simulink model "svm_tracking_1pred_sim"  (Simulink 8.6)
settings: Solver=VariableStepAuto  StartTime=0.0  StopTime=20  RelTol=1e-3
values from neighbouring files (symbols this model uses):
  K = ss(Ttuned.Blocks.K)    [svm_buildLinearControllers.m]
  My = ss(tf([eye(6) -eye(6)]))    [svm_buildLinearControllers.m]
  Mz = ss(tf([pickP, -pickP]))    [svm_buildLinearControllers.m]
  turbulence2loadfactors = blkdiag(T_w2nx, T_w2nz)    [svm_buildLinearControllers.m]
  uavsim = loaded.uavsim    [svm_sandbox.m]
  x0 = history(1).u_apst    [dsmc_extrinsic.m]    (also in svm_buildLinearControllers.m = [0 0 0 0 0 1 0 0 ])
undefined symbols (not defined in the file or in its folder): F, Light, MIL, sigbuilder_block, uavsimblockset_cartesianToAngle
libraries: aerolibwind2 x1, aerolibgravity2 x1, uavsimBlockset_VectorNorm x1, aerolibtransform2 x1
settings Model: Creator=j.bolting  LastModifiedBy=j.bolting
settings DataIOCC: SaveFormat=StructureWithTime  SignalLoggingSaveFormat=Dataset
settings OptimizationCC: BlockReduction=off  DefaultParameterBehavior=Inlined  BufferReuse=off  ExpressionDepthLimit=128
settings DebuggingCC: AlgebraicLoopMsg=none  UnderspecifiedInitializationDetection=Simplified  MergeDetectMultiDrivingBlocksExec=error  SolverPrmCheckMsg=none  FcnCallInpInsideContextMsg=EnableAllAsError  UnconnectedInputMsg=none  UnconnectedOutputMsg=none  UnconnectedLineMsg=none  StateNameClashWarn=none  InitInArrayFormatMsg=none
settings HardwareCC: ProdBitPerPointer=64  ProdLargestAtomicFloat=Float  ProdIntDivRoundTo=Zero  ProdEndianess=LittleEndian  ProdWordSize=64  ProdHWDeviceType=Intel->x86-64 (Windows64)
settings GRTTargetCC: GeneratePreprocessorConditionals=Use local settings  CombineOutputUpdateFcns=on  GRTInterface=off
settings ConfigComp: CovModelRefEnable=off

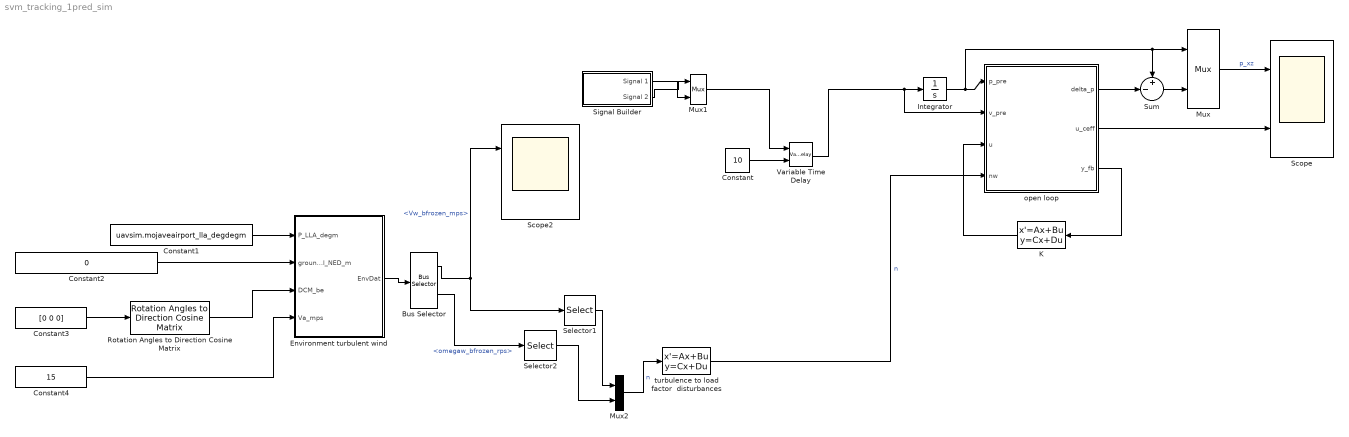
== system svm_tracking_1pred_sim ==
  Bus Selector : BusSelector  OutputSignals=Vw_bfrozen_mps,omegaw_bfrozen_rps
  Constant : Constant  Value=10
  Constant1 : Constant  Value=uavsim.mojaveairport_lla_degdegm
  Constant2 : Constant  Value=0
  Constant3 : Constant  Value=[0 0 0]
  Constant4 : Constant  Value=15
  Environment turbulent wind : Subsystem  AncestorBlock=uavsimBlockset_Environment_turbulentWind/Environment turbulent wind  mask{mask_constantwind_NED_mps=[5 0 0], mask_wingspan=uavsim.cularis.b, mask_windON=0, mask_turbulenceON=1}
      mask prompts: mask_constantwind_NED_mps "Ambient, i.e. constant wind vector [m/s], NED frame"; mask_wingspan "Aircraft wingspan"; mask_windON "Ambient wind ON?"; mask_turbulenceON "Turbulence ON?"
  Integrator : Integrator
  K : StateSpace  A=K.a  B=K.b  C=K.c  D=K.d  X0=0
  Mux : Mux  Inputs=2
  Mux1 : Mux  Inputs=2
  Mux2 : Mux  Inputs=2
  Rotation Angles to Direction Cosine Matrix : aerolibtransform2/Rotation Angles to Direction Cosine Matrix  rotationOrder=ZYX
  Scope : Scope  NumInputPorts=2
  Scope2 : Scope  NumInputPorts=2
  Selector1 : Selector  InputPortWidth=3  IndexOptions=Index vector (dialog)  Indices=[1 3]  OutputSizes=1
  Selector2 : Selector  InputPortWidth=3  IndexOptions=Index vector (dialog)  Indices=2  OutputSizes=1
  Signal Builder : Subsystem  Tag=STV Subsys  LoadFcn=sigbuilder_block('load');  StartFcn=sigbuilder_block('start');  StopFcn=sigbuilder_block('stop');  ClipboardFcn=sigbuilder_block('clipboard');  mask(Sigbuilder block){}
      mask help: Simulink:masks:SigbuilderBlock_MD
      mask init:
      | if ~strcmp(get_param(bdroot(gcbh),'SimulationStatus'),'stopped') tuvar = sigbuilder_block('maskInit'); end
      settings: CopyFcn=sigbuilder_block('copy');  DeleteFcn=sigbuilder_block('delete');  ModelCloseFcn=sigbuilder_block('modelClose');  PreSaveFcn=sigbuilder_block('preSave');  PauseFcn=sigbuilder_block('pause');  ContinueFcn=sigbuilder_block('continue');  NameChangeFcn=sigbuilder_block('namechange');  OpenFcn=sigbuilder_block('open',[437.6 199.2 550.4 400 ]);  CloseFcn=sigbuilder_block('close');
      mask Display: plot(0, 0, 100, 100,[2, 2, 32, 32, 2], [68, 8, 8, 68, 68],[32, 2], [38, 38], [32, 19, 2],[53, 60, 44], [32, 17, 17, 2],[16, 16, 31, 31]);txt = getActiveGroup(gcbh);text(2, 100, txt,'verticalAlignment', 'top');
  Sum : Sum  Inputs=+-|
  Variable Time Delay : VariableTransportDelay  MaximumDelay=1e3
  open loop : Subsystem
  turbulence to load factor  disturbances : StateSpace  A=turbulence2loadfactors.a  B=turbulence2loadfactors.b  C=turbulence2loadfactors.c  D=turbulence2loadfactors.d  X0=0
  wires:
  open loop/3(y_fb) -> K/1
  K/1 -> open loop/3(u)
  open loop/1(delta_p) -> Sum/2
  Sum/1 -> Mux/2
  Variable Time Delay/1 -> Integrator/1, open loop/2(v_pre)
  Mux/1 -> Scope/1  "p_xz"
  open loop/2(u_ceff) -> Scope/2
  Integrator/1 -> Sum/1, Mux/1, open loop/1(p_pre)
  Signal Builder/1(Signal 1) -> Mux1/2
  Signal Builder/2(Signal 2) -> Mux1/1
  Constant/1 -> Variable Time Delay/2
  Mux1/1 -> Variable Time Delay/1
  Environment turbulent wind/1(EnvDat) -> Bus Selector/1
  Bus Selector/1 -> Selector1/1, Scope2/1  "<Vw_bfrozen_mps>"
  Constant1/1 -> Environment turbulent wind/1(P_LLA_degm)
  Constant2/1 -> Environment turbulent wind/2(groundlevel_NED_m)
  Rotation Angles to Direction Cosine Matrix/1 -> Environment turbulent wind/3(DCM_be)
  Constant3/1 -> Rotation Angles to Direction Cosine Matrix/1
  Constant4/1 -> Environment turbulent wind/4(Va_mps)
  Bus Selector/2 -> Selector2/1  "<omegaw_bfrozen_rps>"
  Selector1/1 -> Mux2/1
  Selector2/1 -> Mux2/2
  Mux2/1 -> turbulence to load factor  disturbances/1  "n"
  turbulence to load factor  disturbances/1 -> open loop/4(nw)  "n"

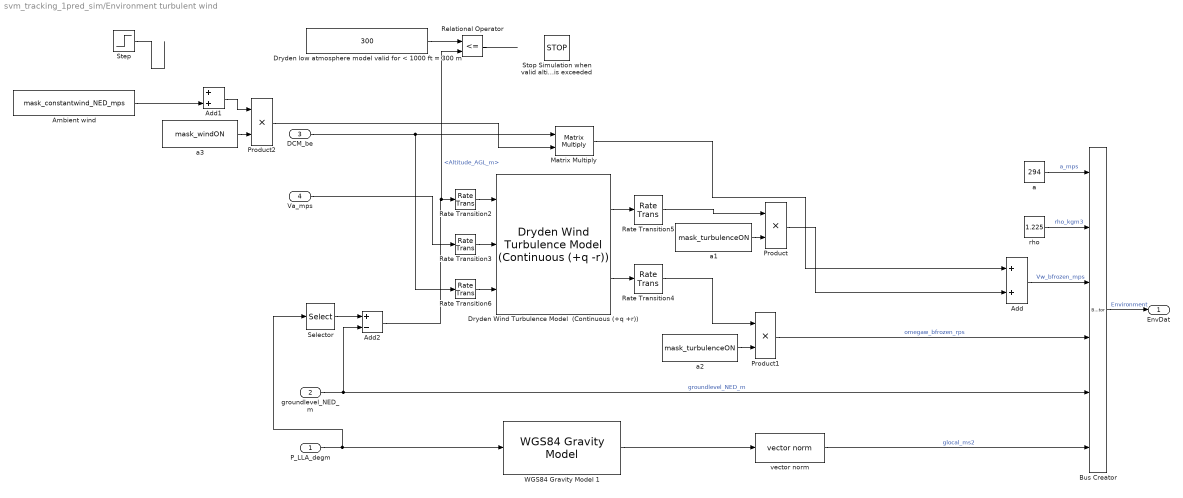
== system svm_tracking_1pred_sim/Environment turbulent wind ==
  P_LLA_degm : Inport
  groundlevel_NED_m : Inport  Port=2
  DCM_be : Inport  Port=3
  Va_mps : Inport  Port=4
  Add : Sum
  Add1 : Sum
  Add2 : Sum  Inputs=+-
  Ambient wind : Constant  Value=mask_constantwind_NED_mps
  Bus Creator : BusCreator  Inputs=6  OutDataTypeStr=Bus: Environment  NonVirtualBus=on
  Dryden Wind Turbulence Model  (Continuous (+q +r)) : aerolibwind2/Dryden Wind Turbulence Model  (Continuous (+q -r))  units=Metric (MKS)  spec=MIL-F-8785C  model=Discrete Dryden (+q -r)  W20=norm(mask_constantwind_NED_mps)  Wdeg=rad2deg(uavsimblockset_cartesianToAngle(mask_constantwind_NED_mps(1), mask_constantwind_NED_mps(2)))  TurbProb=10^-2 - Light  L_high=533.4  Wingspan=mask_wingspan  ts=0.1  Seed=randi(2^6, [1 4])  T_on=on
  Dryden low atmosphere model valid for < 1000 ft = 300 m : Constant  Value=300
  Matrix Multiply : Product  Multiplication=Matrix(*)
  Product : Product  RndMeth=Zero
  Product1 : Product  RndMeth=Zero
  Product2 : Product  RndMeth=Zero
  Rate Transition2 : RateTransition  OutPortSampleTime=0.1
  Rate Transition3 : RateTransition  OutPortSampleTime=0.1
  Rate Transition4 : RateTransition  OutPortSampleTime=0
  Rate Transition5 : RateTransition  OutPortSampleTime=0
  Rate Transition6 : RateTransition  OutPortSampleTime=0.1
  Relational Operator : RelationalOperator  Operator=<=  OutDataTypeStr=boolean
  Selector : Selector  InputPortWidth=3  IndexOptions=Index vector (dialog)  Indices=3  OutputSizes=1
  Step : Step  Time=10  After=[0 0 1]  SampleTime=0
  Stop Simulation when valid altitude is exceeded : Stop
  WGS84 Gravity Model 1 : aerolibgravity2/WGS84 Gravity Model   model=WGS84 Taylor Series  units=Metric (MKS)  no_atmos=on  precessing=on  jd_loc=off  month=October  day=10  year=2004  no_centrifugal=on  action=Warning
  a : Constant  Value=294
  a1 : Constant  Value=mask_turbulenceON
  a2 : Constant  Value=mask_turbulenceON
  a3 : Constant  Value=mask_windON
  "rho " : Constant  Value=1.225
  vector norm : uavsimBlockset_VectorNorm/vector norm
  EnvDat : Outport  OutDataTypeStr=Bus: Environment
  wires:
  Step/1 -> ?
  Add1/1 -> Product2/1
  Product2/1 -> Matrix Multiply/2
  a3/1 -> Product2/2
  Relational Operator/1 -> ?
  Dryden low atmosphere model valid for < 1000 ft = 300 m/1 -> Relational Operator/1
  Product1/1 -> Bus Creator/4  "omegaw_bfrozen_rps"
  a2/1 -> Product1/2
  a1/1 -> Product/2
  Product/1 -> Add/2
  Dryden Wind Turbulence Model  (Continuous (+q +r))/2 -> Rate Transition4/1
  P_LLA_degm/1 -> WGS84 Gravity Model 1/1, Selector/1
  groundlevel_NED_m/1 -> Add2/2, Bus Creator/5  "groundlevel_NED_m"
  WGS84 Gravity Model 1/1 -> vector norm/1
  Bus Creator/1 -> EnvDat/1  "Environment"
  "rho "/1 -> Bus Creator/2  "rho_kgm3"
  a/1 -> Bus Creator/1  "a_mps"
  Add/1 -> Bus Creator/3  "Vw_bfrozen_mps"
  vector norm/1 -> Bus Creator/6  "glocal_ms2"
  Add2/1 -> Rate Transition2/1, Relational Operator/2  "<Altitude_AGL_m>"
  Va_mps/1 -> Rate Transition3/1
  DCM_be/1 -> Matrix Multiply/1, Rate Transition6/1
  Ambient wind/1 -> Add1/2
  Dryden Wind Turbulence Model  (Continuous (+q +r))/1 -> Rate Transition5/1
  Matrix Multiply/1 -> Add/1
  Rate Transition4/1 -> Product1/1
  Rate Transition5/1 -> Product/1
  Selector/1 -> Add2/1
  Rate Transition2/1 -> Dryden Wind Turbulence Model  (Continuous (+q +r))/1
  Rate Transition3/1 -> Dryden Wind Turbulence Model  (Continuous (+q +r))/2
  Rate Transition6/1 -> Dryden Wind Turbulence Model  (Continuous (+q +r))/3

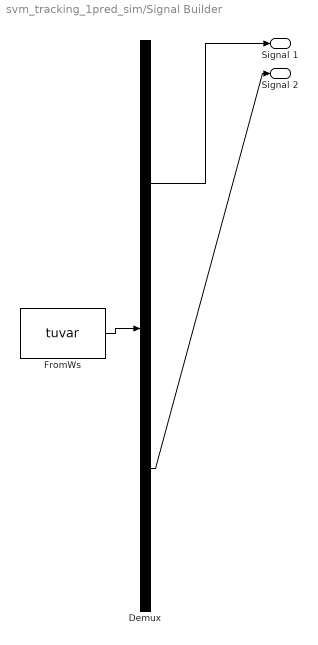
== system svm_tracking_1pred_sim/Signal Builder ==
  Demux : Demux  Tag=STV Demux  Outputs=2
  FromWs : FromWorkspace  Tag=STV FromWs  VariableName=tuvar  SampleTime=0  SigBuilderData=DataTag0  VnvData=DataTag1
      SigBuilderData=|
      | common.afterFinalStr = 'Extrapolate'
      | common.sampleTime = 0
      | dataSet.timeRange = [0 10]
      | dataSet.name = 'Group 1'
      | sbobj.Groups.Name = 'Group 1'
      | sbobj.Groups.Signals(1).Name = 'Signal 1'
      | sbobj.Groups.Signals(1).XData = [0 1.98 1.98 10]
      | sbobj.Groups.Signals(1).YData = [1 1 0 0.01]
      | sbobj.Groups.Signals(2).Name = 'Signal 2'
      | sbobj.Groups.Signals(2).XData = [0 4 6 10]
      | sbobj.Groups.Signals(2).YData = [0 0 0 0]
  Signal 1 : Outport  Tag=STV Outport
  Signal 2 : Outport  Tag=STV Outport  Port=2
  wires:
  Demux/1 -> Signal 1/1
  FromWs/1 -> Demux/1
  Demux/2 -> Signal 2/1

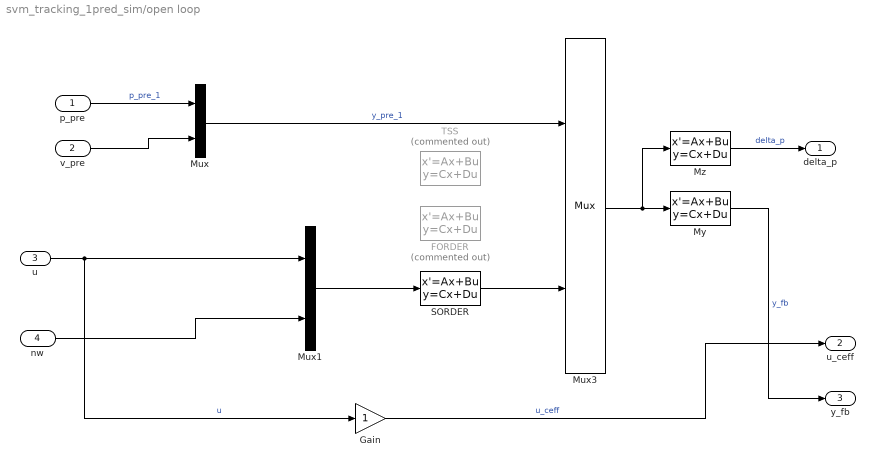
== system svm_tracking_1pred_sim/open loop ==
  p_pre : Inport  PortDimensions=2
  v_pre : Inport  Port=2  PortDimensions=2
  u : Inport  Port=3  PortDimensions=2
  nw : Inport  Port=4  PortDimensions=2
  FORDER : StateSpace  Commented=on  A=uavsim.svm.linearmodels.forder.airspeed_15.a  B=uavsim.svm.linearmodels.forder.airspeed_15.b  C=uavsim.svm.linearmodels.forder.airspeed_15.c  D=uavsim.svm.linearmodels.forder.airspeed_15.d  X0=0
  Gain : Gain
  Mux : Mux  Inputs=2
  Mux1 : Mux  Inputs=2
  Mux3 : Mux  Inputs=2
  My : StateSpace  A=My.a  B=My.b  C=My.c  D=My.d  X0=0
  Mz : StateSpace  A=Mz.a  B=Mz.b  C=Mz.c  D=Mz.d  X0=0
  SORDER : StateSpace  A=uavsim.svm.linearmodels.sorder_longi.airspeed_15.a  B=uavsim.svm.linearmodels.sorder_longi.airspeed_15.b  C=uavsim.svm.linearmodels.sorder_longi.airspeed_15.c  D=uavsim.svm.linearmodels.sorder_longi.airspeed_15.d  X0=x0
  TSS : StateSpace  Commented=on  A=uavsim.svm.linearmodels_tss.airspeed_15.a  B=uavsim.svm.linearmodels_tss.airspeed_15.b  C=uavsim.svm.linearmodels_tss.airspeed_15.c  D=uavsim.svm.linearmodels_tss.airspeed_15.d  X0=0
  delta_p : Outport
  u_ceff : Outport  Port=2
  y_fb : Outport  Port=3
  wires:
  v_pre/1 -> Mux/2
  p_pre/1 -> Mux/1  "p_pre_1"
  Mux/1 -> Mux3/1  "y_pre_1"
  SORDER/1 -> Mux3/2
  Mux3/1 -> Mz/1, My/1
  Mz/1 -> delta_p/1  "delta_p"
  My/1 -> y_fb/1  "y_fb"
  u/1 -> Gain/1, Mux1/1  "u"
  Mux1/1 -> SORDER/1
  Gain/1 -> u_ceff/1  "u_ceff"
  nw/1 -> Mux1/2
